simulink model "series"  (R2018b)
settings: Solver=ode1  StartTime=0.0  StopTime=t_stop  FixedStep=t_sample  RelTol=1e-3
values from neighbouring files (symbols this model uses):
  air_density_sea_level = 1.225    [hybrid_truck_script.m]
  battery_capacity = 24.5    [hybrid_truck_script.m]
  battery_efficiency = 0.8    [hybrid_truck_script.m]
  battery_max_power_flow = battery_v*battery_max_i    (= 23040)    [hybrid_truck_script.m]
  battery_no_of_modules = 15    [hybrid_truck_script.m]
  battery_SoC = 0.95    [hybrid_truck_script.m]
  constant_velocity = 60    [hybrid_truck_script.m]
  distance = 0.20    (= 0.2)    [hybrid_truck_script.m]
  drag_coeff = 0.65    [hybrid_truck_script.m]
  elevation = route.data(:,3)    [hybrid_truck_script.m]
  engine_optimum_rad = engine_rad(engine_optimum_index)    [hybrid_truck_script.m]
  engine_optimum_torque = max(engine_torque)    [hybrid_truck_script.m]
  frontal_area = 5.14    [hybrid_truck_script.m]
  fuel_map = (3.6e6/(engine_efficiency*fuel_LHV*fuel_density))*            (rps_axes'*torque_axes)    [hybrid_truck_script.m]
  g = 9.81    [hybrid_truck_script.m]
  gearRatio_differential = 4.263    [hybrid_truck_script.m]
  gradients = (pi/400).*route.data(:,5)    [hybrid_truck_script.m]
  momentOfInertia_engine = 2.55    [hybrid_truck_script.m]
  momentOfInertia_wheel = 2.5    [hybrid_truck_script.m]
  motor_efficiency = motor(1)    [hybrid_truck_script.m]
  mpsToKPH = 3.6    [hybrid_truck_script.m]
  radius_wheel = 0.46    [hybrid_truck_script.m]
  regeneration_efficiency = 0.75    [hybrid_truck_script.m]
  rolling_resistance = 0.008    [hybrid_truck_script.m]
  rps_axes = linspace(min(engine_rad),max(engine_rad),n)    [hybrid_truck_script.m]
  selection = number associated with the drive cycle (see    [drop_bars.m]    (also in hybrid_truck_script.m = listdlg('ListString', drive_cycle))
  t_sample = 0.1    [hybrid_truck_script.m]
  torque_axes = linspace(min(engine_torque),max(engine_torque),n)    [hybrid_truck_script.m]
  total_mass = mass_truck + mass_trailor    (= 39150)    [hybrid_truck_script.m]
libraries: dspstat3 x1, autolibshared x1
settings Model: Creator=tumisang  LastModifiedBy=tumisang

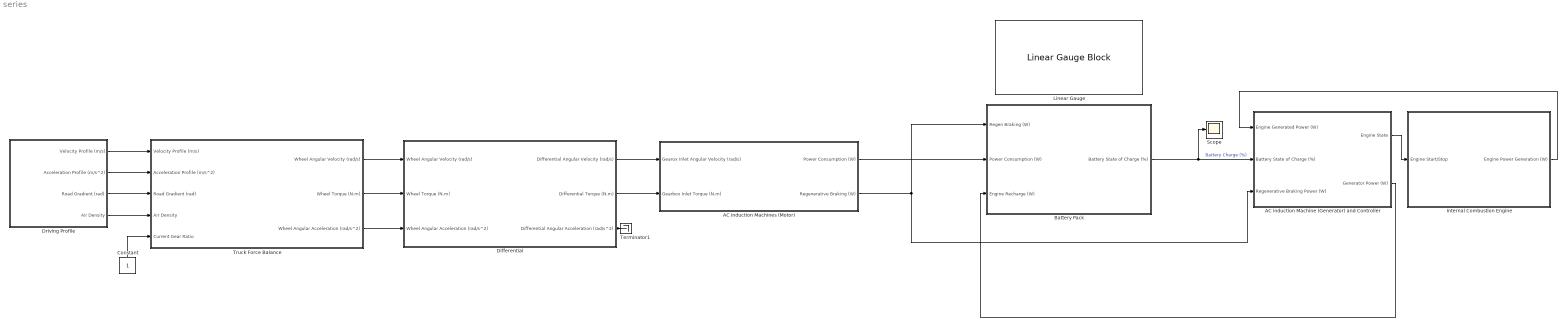
== system series ==
  " Battery Pack" : Subsystem
  AC Induction Machines (Motor) : Subsystem
  AC induction Machine (Generator) and Controller : Subsystem
  Constant : Constant
  Differential : Subsystem
  Driving Profile : Subsystem
  Internal Combustion Engine : Subsystem
  Linear Gauge : LinearGaugeBlock  WebBlockId=520
  Scope : Scope
  Terminator1 : Terminator
  Truck Force Balance : Subsystem
  wires:
  Differential/2(Differential Torque (N.m)) -> AC Induction Machines (Motor)/2(Gearbox Inlet Torque (N.m))
  AC Induction Machines (Motor)/2(Regenerative Braking (W)) -> " Battery Pack"/1(Regen Braking (W)), AC induction Machine (Generator) and Controller/3(Regenerative Braking Power (W))
  Internal Combustion Engine/1(Engine Power Generation (W)) -> AC induction Machine (Generator) and Controller/1(Engine Generated Power (W))
  AC induction Machine (Generator) and Controller/1(Engine State) -> Internal Combustion Engine/1(Engine Start/Stop)
  " Battery Pack"/1(Battery State of Charge (%)) -> AC induction Machine (Generator) and Controller/2(Battery State of Charge (%)), Scope/1  "Battery Charge (%)"
  AC Induction Machines (Motor)/1(Power Consumption (W)) -> " Battery Pack"/2(Power Consumption (W))
  AC induction Machine (Generator) and Controller/2(Generator Power (W)) -> " Battery Pack"/3(Engine Recharge (W))
  Truck Force Balance/3(Wheel Angular Acceleration (rad/s^2)) -> Differential/3(Wheel Angular Acceleration (rad/s^2))
  Truck Force Balance/2(Wheel Torque (N.m)) -> Differential/2(Wheel Torque (N.m))
  Truck Force Balance/1(Wheel Angular Velocity (rad/s)) -> Differential/1(Wheel Angular Velocity (rad/s))
  Constant/1 -> Truck Force Balance/5(Current Gear Ratio)
  Driving Profile/4(Air Density) -> Truck Force Balance/4(Air Density)
  Driving Profile/2(Acceleration Profile (m/s^2)) -> Truck Force Balance/2(Acceleration Profile (m/s^2))
  Driving Profile/1(Velocity Profile (m/s)) -> Truck Force Balance/1(Velocity Profile (m/s))
  Driving Profile/3(Road Gradient (rad)) -> Truck Force Balance/3(Road Gradient (rad))
  Differential/1(Differential Angular Velocity (rad/s)) -> AC Induction Machines (Motor)/1(Gearox Inlet Angular Velocity (rad/s))
  Differential/3(Differential Angular Acceleration (rad/s^2)) -> Terminator1/1

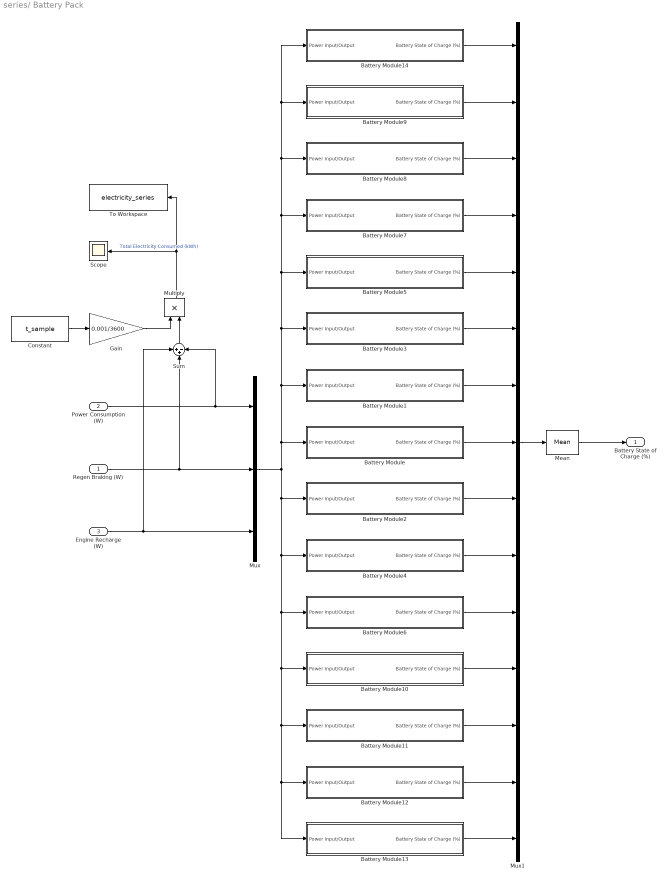
== system series/ Battery Pack ==
  Regen Braking (W) : Inport
  Power Consumption (W) : Inport  Port=2
  Engine Recharge (W) : Inport  Port=3
  Battery Module : Subsystem
  Battery Module1 : Subsystem
  Battery Module10 : Subsystem
  Battery Module11 : Subsystem
  Battery Module12 : Subsystem
  Battery Module13 : Subsystem
  Battery Module14 : Subsystem
  Battery Module2 : Subsystem
  Battery Module3 : Subsystem
  Battery Module4 : Subsystem
  Battery Module5 : Subsystem
  Battery Module6 : Subsystem
  Battery Module7 : Subsystem
  Battery Module8 : Subsystem
  Battery Module9 : Subsystem
  Constant : Constant  Value=t_sample
  Gain : Gain  Gain=0.001/3600
  Mean : dspstat3/Mean  run=off  InputProcessing=Columns as channels (frame based)  reset_popup=None  directionMode=Each column  dimension=1  roiEnable=off  roiType=Rectangles  roiPortion=Entire ROI  roiOutput=Individual statistics for each ROI  roiFlag=off  roundingMode=Floor  overflowMode=off  outputDataTypeStr=Inherit: Same as accumulator  outputMin=[]  outputMax=[]  outputLastDataTypeStr=Inherit: Same as accumulator
  Multiply : Product
  Mux : Mux  Inputs=3
  Mux1 : Mux  Inputs=15
  Scope : Scope
  Sum : Sum  Inputs=++-
  To Workspace : ToWorkspace  VariableName=electricity_series  SaveFormat=Timeseries  SampleTime=-1
  Battery State of Charge (%) : Outport
  wires:
  Mux/1 -> Battery Module11/1(Power Input/Output), Battery Module12/1(Power Input/Output), Battery Module13/1(Power Input/Output), Battery Module10/1(Power Input/Output), Battery Module6/1(Power Input/Output), Battery Module4/1(Power Input/Output), Battery Module2/1(Power Input/Output), Battery Module5/1(Power Input/Output), Battery Module7/1(Power Input/Output), Battery Module8/1(Power Input/Output), Battery Module9/1(Power Input/Output), Battery Module14/1(Power Input/Output), Battery Module3/1(Power Input/Output), Battery Module1/1(Power Input/Output), Battery Module/1(Power Input/Output)
  Battery Module1/1(Battery State of Charge (%)) -> Mux1/7
  Battery Module/1(Battery State of Charge (%)) -> Mux1/8
  Battery Module2/1(Battery State of Charge (%)) -> Mux1/9
  Battery Module4/1(Battery State of Charge (%)) -> Mux1/10
  Battery Module6/1(Battery State of Charge (%)) -> Mux1/11
  Battery Module3/1(Battery State of Charge (%)) -> Mux1/6
  Battery Module5/1(Battery State of Charge (%)) -> Mux1/5
  Battery Module7/1(Battery State of Charge (%)) -> Mux1/4
  Battery Module8/1(Battery State of Charge (%)) -> Mux1/3
  Battery Module9/1(Battery State of Charge (%)) -> Mux1/2
  Battery Module14/1(Battery State of Charge (%)) -> Mux1/1
  Battery Module10/1(Battery State of Charge (%)) -> Mux1/12
  Battery Module11/1(Battery State of Charge (%)) -> Mux1/13
  Battery Module12/1(Battery State of Charge (%)) -> Mux1/14
  Battery Module13/1(Battery State of Charge (%)) -> Mux1/15
  Mean/1 -> Battery State of Charge (%)/1
  Mux1/1 -> Mean/1
  Engine Recharge (W)/1 -> Mux/3, Sum/1
  Constant/1 -> Gain/1
  Power Consumption (W)/1 -> Mux/1, Sum/3
  Sum/1 -> Multiply/2
  Multiply/1 -> Scope/1, To Workspace/1  "Total Electricity Consumed (kWh)"
  Regen Braking (W)/1 -> Sum/2, Mux/2
  Gain/1 -> Multiply/1

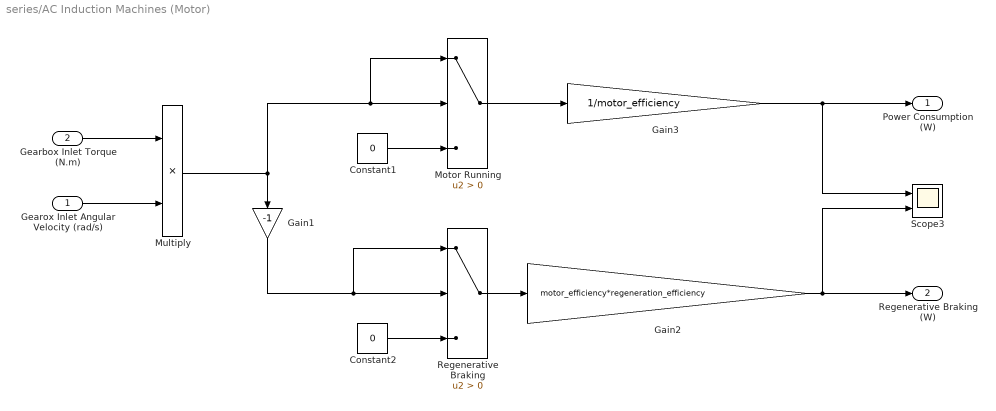
== system series/AC Induction Machines (Motor) ==
  Gearox Inlet Angular Velocity (rad/s) : Inport
  Gearbox Inlet Torque (N.m) : Inport  Port=2
  Constant1 : Constant  Value=0
  Constant2 : Constant  Value=0
  Gain1 : Gain  Gain=-1
  Gain2 : Gain  Gain=motor_efficiency*regeneration_efficiency
  Gain3 : Gain  Gain=1/motor_efficiency
  Motor Running : Switch  Criteria=u2 > Threshold
  Multiply : Product
  Regenerative Braking : Switch  Criteria=u2 > Threshold
  Scope3 : Scope  NumInputPorts=2
  Power Consumption (W) : Outport
  Regenerative Braking (W) : Outport  Port=2
  wires:
  Constant2/1 -> Regenerative Braking/3
  Constant1/1 -> Motor Running/3
  Gain2/1 -> Regenerative Braking (W)/1, Scope3/2
  Regenerative Braking/1 -> Gain2/1
  Multiply/1 -> Gain1/1, Motor Running/2, Motor Running/1
  Gain3/1 -> Power Consumption (W)/1, Scope3/1
  Gearox Inlet Angular Velocity (rad/s)/1 -> Multiply/2
  Gearbox Inlet Torque (N.m)/1 -> Multiply/1
  Motor Running/1 -> Gain3/1
  Gain1/1 -> Regenerative Braking/1, Regenerative Braking/2

== system series/AC induction Machine (Generator) and Controller ==
  Engine Generated Power (W) : Inport
  Battery State of Charge (%) : Inport  Port=2
  Regenerative Braking Power (W) : Inport  Port=3
  Engine On/Off Logic : Stateflow chart  TreatAsAtomicUnit=on
  Gain2 : Gain  Gain=regeneration_efficiency
  Engine State : Outport
  Generator Power (W) : Outport  Port=2
  wires:
  Gain2/1 -> Generator Power (W)/1
  Regenerative Braking Power (W)/1 -> Engine On/Off Logic/2(regen_power)
  Engine Generated Power (W)/1 -> Gain2/1
  Engine On/Off Logic/1(state) -> Engine State/1
  Battery State of Charge (%)/1 -> Engine On/Off Logic/1(battery_SoC)

== system series/Differential ==
  Wheel Angular Velocity (rad/s) : Inport
  Wheel Torque (N.m) : Inport  Port=2
  Wheel Angular Acceleration (rad/s^2) : Inport  Port=3
  Gain1 : Gain  Gain=1/gearRatio_differential
  Gain2 : Gain  Gain=gearRatio_differential
  Gain3 : Gain  Gain=gearRatio_differential
  Differential Angular Velocity (rad/s) : Outport
  Differential Torque (N.m) : Outport  Port=2
  Differential Angular Acceleration (rad/s^2) : Outport  Port=3
  wires:
  Gain2/1 -> Differential Angular Acceleration (rad/s^2)/1
  Gain3/1 -> Differential Angular Velocity (rad/s)/1
  Wheel Angular Acceleration (rad/s^2)/1 -> Gain2/1
  Wheel Torque (N.m)/1 -> Gain1/1
  Gain1/1 -> Differential Torque (N.m)/1
  Wheel Angular Velocity (rad/s)/1 -> Gain3/1

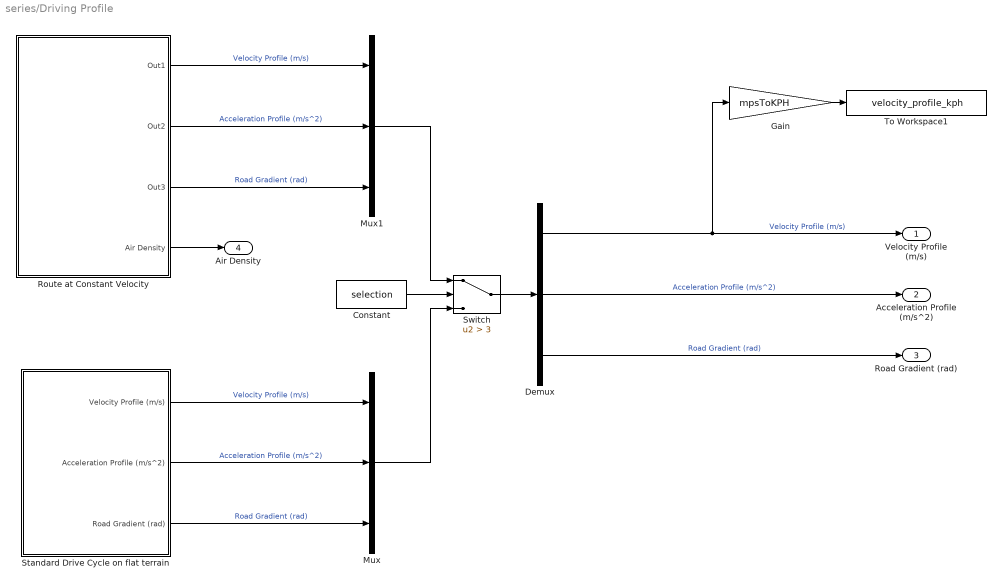
== system series/Driving Profile ==
  Constant : Constant  Value=selection
  Demux : Demux  Outputs=3
  Gain : Gain  Gain=mpsToKPH
  Mux : Mux  Inputs=3
  Mux1 : Mux  Inputs=3
  Route at Constant Velocity : Subsystem
  Standard Drive Cycle on flat terrain : Subsystem
  Switch : Switch  Criteria=u2 > Threshold  Threshold=3
  To Workspace1 : ToWorkspace  VariableName=velocity_profile_kph  SaveFormat=Timeseries  SampleTime=-1
  Velocity Profile (m/s) : Outport
  Acceleration Profile (m/s^2) : Outport  Port=2
  Road Gradient (rad) : Outport  Port=3
  Air Density : Outport  Port=4
  wires:
  Route at Constant Velocity/3(Out3) -> Mux1/3  "Road Gradient (rad)"
  Route at Constant Velocity/2(Out2) -> Mux1/2  "Acceleration Profile (m/s^2)"
  Demux/1 -> Velocity Profile (m/s)/1, Gain/1  "Velocity Profile (m/s)"
  Standard Drive Cycle on flat terrain/2(Acceleration Profile (m/s^2)) -> Mux/2  "Acceleration Profile (m/s^2)"
  Demux/2 -> Acceleration Profile (m/s^2)/1  "Acceleration Profile (m/s^2)"
  Standard Drive Cycle on flat terrain/3(Road Gradient (rad)) -> Mux/3  "Road Gradient (rad)"
  Demux/3 -> Road Gradient (rad)/1  "Road Gradient (rad)"
  Route at Constant Velocity/1(Out1) -> Mux1/1  "Velocity Profile (m/s)"
  Standard Drive Cycle on flat terrain/1(Velocity Profile (m/s)) -> Mux/1  "Velocity Profile (m/s)"
  Gain/1 -> To Workspace1/1
  Constant/1 -> Switch/2
  Switch/1 -> Demux/1
  Mux/1 -> Switch/3
  Mux1/1 -> Switch/1
  Route at Constant Velocity/4(Air Density) -> Air Density/1

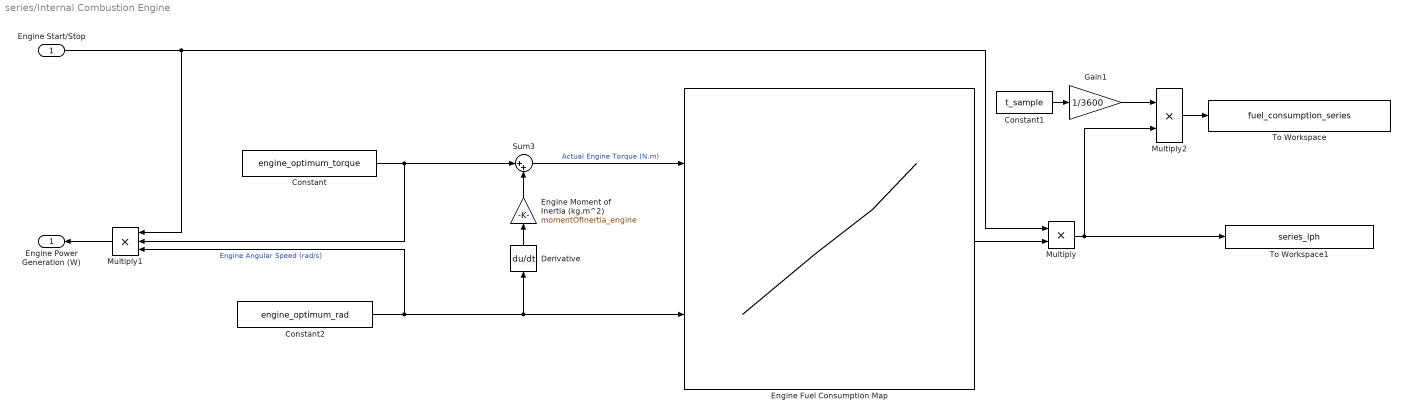
== system series/Internal Combustion Engine ==
  Engine Start/Stop : Inport
  Constant : Constant  Value=engine_optimum_torque
  Constant1 : Constant  Value=t_sample
  Constant2 : Constant  Value=engine_optimum_rad
  Derivative : Derivative  CoefficientInTFapproximation=0
  Engine Fuel Consumption Map : Lookup_n-D  BreakpointsForDimension1=torque_axes  BreakpointsForDimension2=rps_axes  Table=fuel_map  InternalRulePriority=Speed  RndMeth=Simplest  InputSameDT=on
  Engine Moment of Inertia (kg.m^2) : Gain  Gain=momentOfInertia_engine
  Gain1 : Gain  Gain=1/3600
  Multiply : Product
  Multiply1 : Product  Inputs=3
  Multiply2 : Product
  Sum3 : Sum  Inputs=|++
  To Workspace : ToWorkspace  VariableName=fuel_consumption_series  SaveFormat=Timeseries  SampleTime=-1
  To Workspace1 : ToWorkspace  VariableName=series_lph  SaveFormat=Timeseries  SampleTime=-1
  Engine Power Generation (W) : Outport
  wires:
  Constant2/1 -> Engine Fuel Consumption Map/2, Derivative/1, Multiply1/3  "Engine Angular Speed (rad/s)"
  Sum3/1 -> Engine Fuel Consumption Map/1  "Actual Engine Torque (N.m)"
  Engine Moment of Inertia (kg.m^2)/1 -> Sum3/2
  Engine Fuel Consumption Map/1 -> Multiply/2
  Derivative/1 -> Engine Moment of Inertia (kg.m^2)/1
  Constant/1 -> Multiply1/2, Sum3/1
  Engine Start/Stop/1 -> Multiply/1, Multiply1/1
  Multiply1/1 -> Engine Power Generation (W)/1
  Multiply/1 -> To Workspace1/1, Multiply2/2
  Multiply2/1 -> To Workspace/1
  Gain1/1 -> Multiply2/1
  Constant1/1 -> Gain1/1

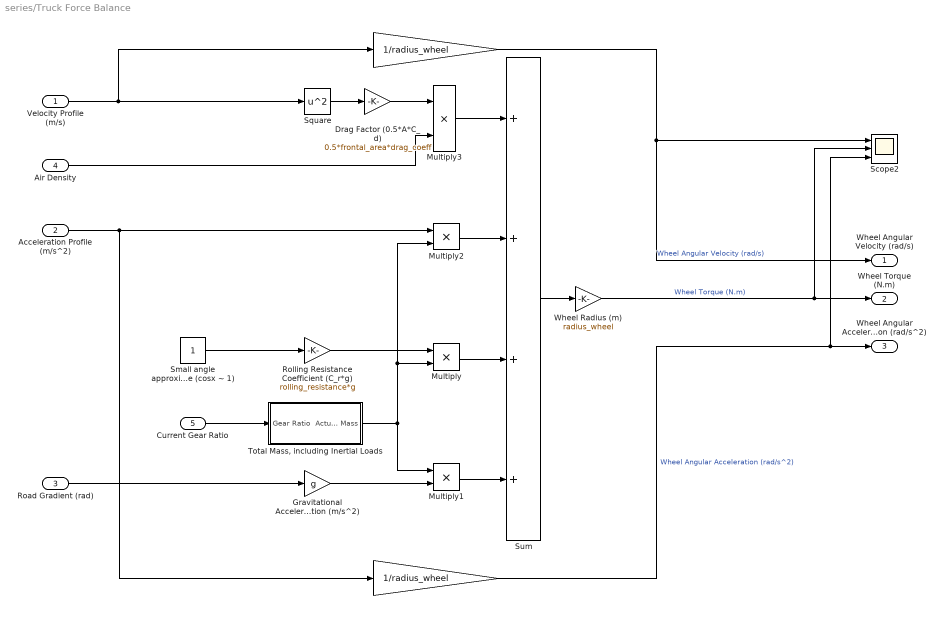
== system series/Truck Force Balance ==
  Velocity Profile (m/s) : Inport
  Acceleration Profile (m/s^2) : Inport  Port=2
  Road Gradient (rad) : Inport  Port=3
  Air Density : Inport  Port=4
  Current Gear Ratio : Inport  Port=5
  " " : Gain  Gain=1/radius_wheel
  " " : Gain  Gain=1/radius_wheel
  Drag Factor (0.5*A*C_d) : Gain  Gain=0.5*frontal_area*drag_coeff
  Gravitational Acceleration (m/s^2) : Gain  Gain=g
  Multiply{,1..3} (4 alike) : Product
  Rolling Resistance Coefficient (C_r*g) : Gain  Gain=rolling_resistance*g
  Scope2 : Scope  NumInputPorts=3
  Small angle approximation for cosine (cosx ~ 1) : Constant
  Square : Math  Operator=square  SaturateOnIntegerOverflow=on
  Sum : Sum  Inputs=++++
  "Total Mass, including Inertial Loads" : Subsystem
  Wheel Radius (m) : Gain  Gain=radius_wheel
  Wheel Angular Velocity (rad/s) : Outport
  Wheel Torque (N.m) : Outport  Port=2
  Wheel Angular Acceleration (rad/s^2) : Outport  Port=3
  wires:
  Square/1 -> Drag Factor (0.5*A*C_d)/1
  Drag Factor (0.5*A*C_d)/1 -> Multiply3/1
  Road Gradient (rad)/1 -> Gravitational Acceleration (m/s^2)/1
  Gravitational Acceleration (m/s^2)/1 -> Multiply1/2
  Velocity Profile (m/s)/1 -> Square/1, " "/1
  Rolling Resistance Coefficient (C_r*g)/1 -> Multiply/1
  Sum/1 -> Wheel Radius (m)/1
  Wheel Radius (m)/1 -> Wheel Torque (N.m)/1, Scope2/2  "Wheel Torque (N.m)"
  " "/1 -> Scope2/3, Wheel Angular Acceleration (rad/s^2)/1  "Wheel Angular Acceleration (rad/s^2)"
  " "/1 -> Wheel Angular Velocity (rad/s)/1, Scope2/1  "Wheel Angular Velocity (rad/s)"
  Multiply2/1 -> Sum/2
  Small angle approximation for cosine (cosx ~ 1)/1 -> Rolling Resistance Coefficient (C_r*g)/1
  Acceleration Profile (m/s^2)/1 -> " "/1, Multiply2/1
  Current Gear Ratio/1 -> "Total Mass, including Inertial Loads"/1("Gear Ratio ")
  "Total Mass, including Inertial Loads"/1(Actual Mass) -> Multiply1/1, Multiply2/2, Multiply/2
  Multiply/1 -> Sum/3
  Multiply1/1 -> Sum/4
  Air Density/1 -> Multiply3/2
  Multiply3/1 -> Sum/1

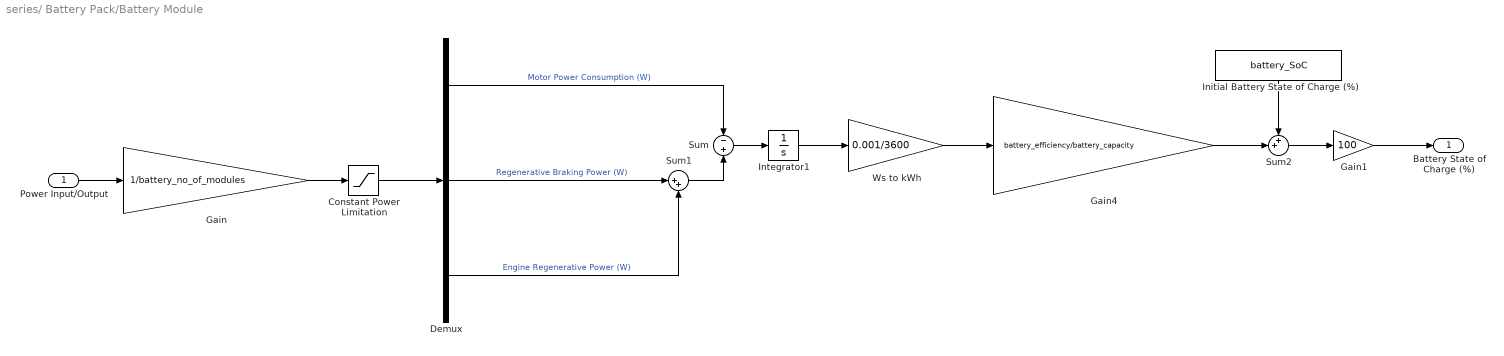
== system series/ Battery Pack/Battery Module ==
  Power Input/Output : Inport
  Constant Power Limitation : Saturate  UpperLimit=battery_max_power_flow  LowerLimit=0
  Demux : Demux  Outputs=3
  Gain : Gain  Gain=1/battery_no_of_modules
  Gain1 : Gain  Gain=100
  Gain4 : Gain  Gain=battery_efficiency/battery_capacity
  Initial Battery State of Charge (%) : Constant  Value=battery_SoC
  Integrator1 : Integrator
  Sum : Sum  Inputs=-+
  Sum1 : Sum  Inputs=|++
  Sum2 : Sum  Inputs=++|
  Ws to kWh : Gain  Gain=0.001/3600
  Battery State of Charge (%) : Outport
  wires:
  Sum/1 -> Integrator1/1
  Ws to kWh/1 -> Gain4/1
  Initial Battery State of Charge (%)/1 -> Sum2/1
  Sum2/1 -> Gain1/1
  Gain1/1 -> Battery State of Charge (%)/1
  Sum1/1 -> Sum/2
  Integrator1/1 -> Ws to kWh/1
  Gain4/1 -> Sum2/2
  Demux/3 -> Sum1/2  "Engine Regenerative Power (W)"
  Demux/2 -> Sum1/1  "Regenerative Braking Power (W)"
  Demux/1 -> Sum/1  "Motor Power Consumption (W)"
  Gain/1 -> Constant Power Limitation/1
  Power Input/Output/1 -> Gain/1
  Constant Power Limitation/1 -> Demux/1

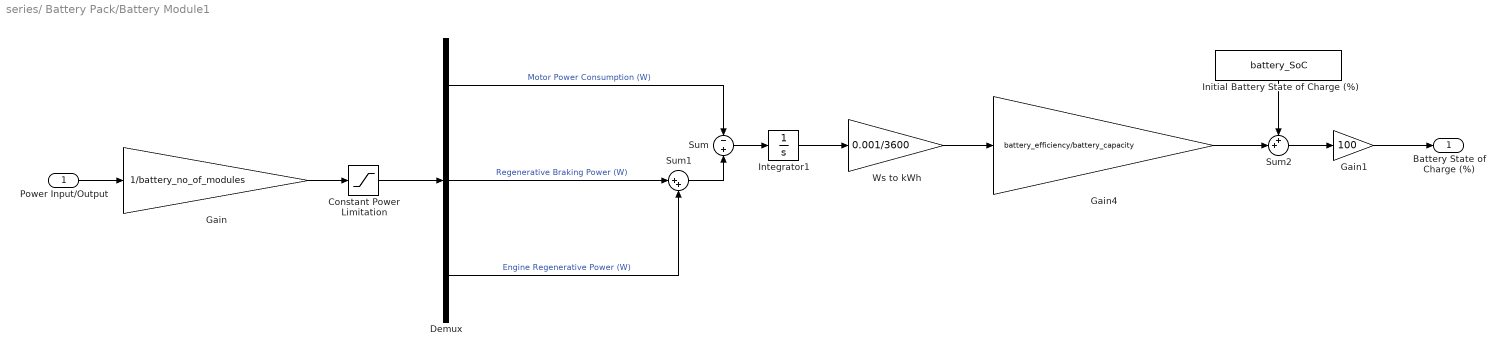
== system series/ Battery Pack/Battery Module1 ==
  Power Input/Output : Inport
  Constant Power Limitation : Saturate  UpperLimit=battery_max_power_flow  LowerLimit=0
  Demux : Demux  Outputs=3
  Gain : Gain  Gain=1/battery_no_of_modules
  Gain1 : Gain  Gain=100
  Gain4 : Gain  Gain=battery_efficiency/battery_capacity
  Initial Battery State of Charge (%) : Constant  Value=battery_SoC
  Integrator1 : Integrator
  Sum : Sum  Inputs=-+
  Sum1 : Sum  Inputs=|++
  Sum2 : Sum  Inputs=++|
  Ws to kWh : Gain  Gain=0.001/3600
  Battery State of Charge (%) : Outport
  wires:
  Constant Power Limitation/1 -> Demux/1
  Power Input/Output/1 -> Gain/1
  Gain/1 -> Constant Power Limitation/1
  Demux/1 -> Sum/1  "Motor Power Consumption (W)"
  Demux/2 -> Sum1/1  "Regenerative Braking Power (W)"
  Demux/3 -> Sum1/2  "Engine Regenerative Power (W)"
  Gain4/1 -> Sum2/2
  Integrator1/1 -> Ws to kWh/1
  Sum1/1 -> Sum/2
  Gain1/1 -> Battery State of Charge (%)/1
  Sum2/1 -> Gain1/1
  Initial Battery State of Charge (%)/1 -> Sum2/1
  Ws to kWh/1 -> Gain4/1
  Sum/1 -> Integrator1/1

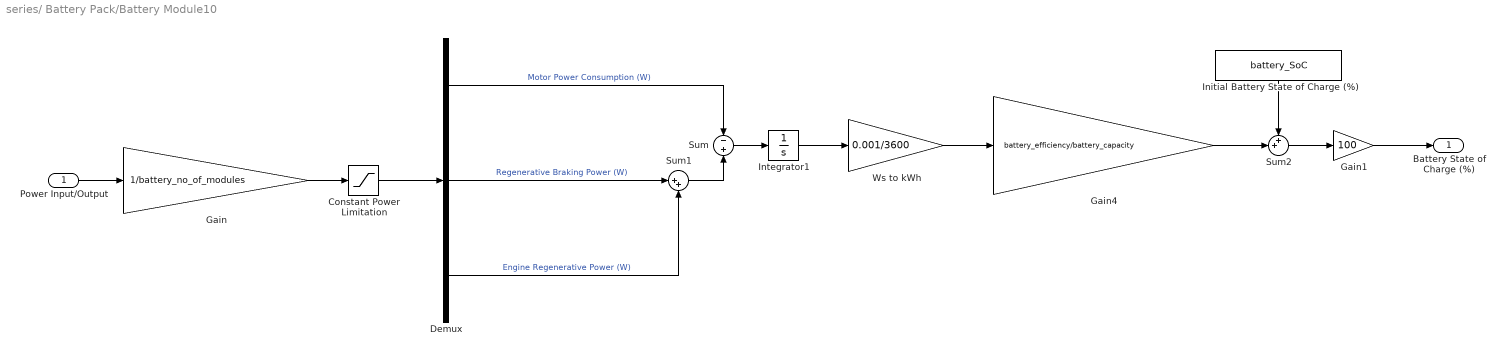
== system series/ Battery Pack/Battery Module10 ==
  Power Input/Output : Inport
  Constant Power Limitation : Saturate  UpperLimit=battery_max_power_flow  LowerLimit=0
  Demux : Demux  Outputs=3
  Gain : Gain  Gain=1/battery_no_of_modules
  Gain1 : Gain  Gain=100
  Gain4 : Gain  Gain=battery_efficiency/battery_capacity
  Initial Battery State of Charge (%) : Constant  Value=battery_SoC
  Integrator1 : Integrator
  Sum : Sum  Inputs=-+
  Sum1 : Sum  Inputs=|++
  Sum2 : Sum  Inputs=++|
  Ws to kWh : Gain  Gain=0.001/3600
  Battery State of Charge (%) : Outport
  wires:
  Constant Power Limitation/1 -> Demux/1
  Power Input/Output/1 -> Gain/1
  Gain/1 -> Constant Power Limitation/1
  Demux/1 -> Sum/1  "Motor Power Consumption (W)"
  Demux/2 -> Sum1/1  "Regenerative Braking Power (W)"
  Demux/3 -> Sum1/2  "Engine Regenerative Power (W)"
  Gain4/1 -> Sum2/2
  Integrator1/1 -> Ws to kWh/1
  Sum1/1 -> Sum/2
  Gain1/1 -> Battery State of Charge (%)/1
  Sum2/1 -> Gain1/1
  Initial Battery State of Charge (%)/1 -> Sum2/1
  Ws to kWh/1 -> Gain4/1
  Sum/1 -> Integrator1/1

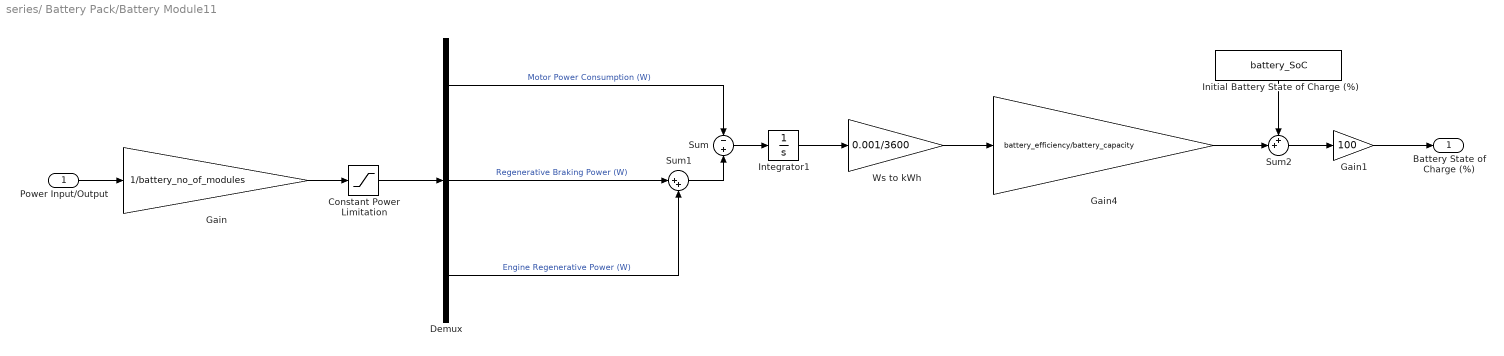
== system series/ Battery Pack/Battery Module11 ==
  Power Input/Output : Inport
  Constant Power Limitation : Saturate  UpperLimit=battery_max_power_flow  LowerLimit=0
  Demux : Demux  Outputs=3
  Gain : Gain  Gain=1/battery_no_of_modules
  Gain1 : Gain  Gain=100
  Gain4 : Gain  Gain=battery_efficiency/battery_capacity
  Initial Battery State of Charge (%) : Constant  Value=battery_SoC
  Integrator1 : Integrator
  Sum : Sum  Inputs=-+
  Sum1 : Sum  Inputs=|++
  Sum2 : Sum  Inputs=++|
  Ws to kWh : Gain  Gain=0.001/3600
  Battery State of Charge (%) : Outport
  wires:
  Sum/1 -> Integrator1/1
  Ws to kWh/1 -> Gain4/1
  Initial Battery State of Charge (%)/1 -> Sum2/1
  Sum2/1 -> Gain1/1
  Gain1/1 -> Battery State of Charge (%)/1
  Sum1/1 -> Sum/2
  Integrator1/1 -> Ws to kWh/1
  Gain4/1 -> Sum2/2
  Demux/3 -> Sum1/2  "Engine Regenerative Power (W)"
  Demux/2 -> Sum1/1  "Regenerative Braking Power (W)"
  Demux/1 -> Sum/1  "Motor Power Consumption (W)"
  Gain/1 -> Constant Power Limitation/1
  Power Input/Output/1 -> Gain/1
  Constant Power Limitation/1 -> Demux/1

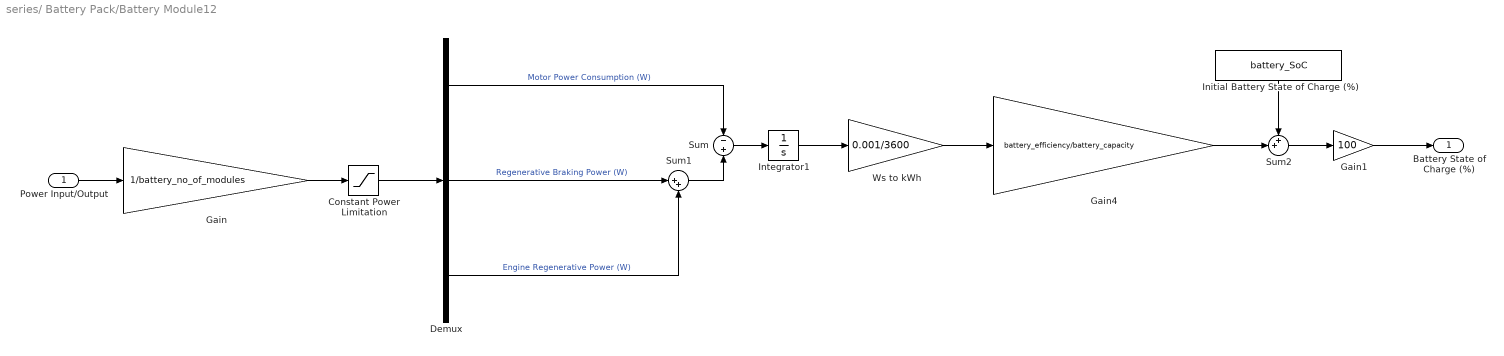
== system series/ Battery Pack/Battery Module12 ==
  Power Input/Output : Inport
  Constant Power Limitation : Saturate  UpperLimit=battery_max_power_flow  LowerLimit=0
  Demux : Demux  Outputs=3
  Gain : Gain  Gain=1/battery_no_of_modules
  Gain1 : Gain  Gain=100
  Gain4 : Gain  Gain=battery_efficiency/battery_capacity
  Initial Battery State of Charge (%) : Constant  Value=battery_SoC
  Integrator1 : Integrator
  Sum : Sum  Inputs=-+
  Sum1 : Sum  Inputs=|++
  Sum2 : Sum  Inputs=++|
  Ws to kWh : Gain  Gain=0.001/3600
  Battery State of Charge (%) : Outport
  wires:
  Constant Power Limitation/1 -> Demux/1
  Power Input/Output/1 -> Gain/1
  Gain/1 -> Constant Power Limitation/1
  Demux/1 -> Sum/1  "Motor Power Consumption (W)"
  Demux/2 -> Sum1/1  "Regenerative Braking Power (W)"
  Demux/3 -> Sum1/2  "Engine Regenerative Power (W)"
  Gain4/1 -> Sum2/2
  Integrator1/1 -> Ws to kWh/1
  Sum1/1 -> Sum/2
  Gain1/1 -> Battery State of Charge (%)/1
  Sum2/1 -> Gain1/1
  Initial Battery State of Charge (%)/1 -> Sum2/1
  Ws to kWh/1 -> Gain4/1
  Sum/1 -> Integrator1/1

== system series/ Battery Pack/Battery Module13 ==
  Power Input/Output : Inport
  Constant Power Limitation : Saturate  UpperLimit=battery_max_power_flow  LowerLimit=0
  Demux : Demux  Outputs=3
  Gain : Gain  Gain=1/battery_no_of_modules
  Gain1 : Gain  Gain=100
  Gain4 : Gain  Gain=battery_efficiency/battery_capacity
  Initial Battery State of Charge (%) : Constant  Value=battery_SoC
  Integrator1 : Integrator
  Sum : Sum  Inputs=-+
  Sum1 : Sum  Inputs=|++
  Sum2 : Sum  Inputs=++|
  Ws to kWh : Gain  Gain=0.001/3600
  Battery State of Charge (%) : Outport
  wires:
  Sum/1 -> Integrator1/1
  Ws to kWh/1 -> Gain4/1
  Initial Battery State of Charge (%)/1 -> Sum2/1
  Sum2/1 -> Gain1/1
  Gain1/1 -> Battery State of Charge (%)/1
  Sum1/1 -> Sum/2
  Integrator1/1 -> Ws to kWh/1
  Gain4/1 -> Sum2/2
  Demux/3 -> Sum1/2  "Engine Regenerative Power (W)"
  Demux/2 -> Sum1/1  "Regenerative Braking Power (W)"
  Demux/1 -> Sum/1  "Motor Power Consumption (W)"
  Gain/1 -> Constant Power Limitation/1
  Power Input/Output/1 -> Gain/1
  Constant Power Limitation/1 -> Demux/1

== system series/ Battery Pack/Battery Module14 ==
  Power Input/Output : Inport
  Constant Power Limitation : Saturate  UpperLimit=battery_max_power_flow  LowerLimit=0
  Demux : Demux  Outputs=3
  Gain : Gain  Gain=1/battery_no_of_modules
  Gain1 : Gain  Gain=100
  Gain4 : Gain  Gain=battery_efficiency/battery_capacity
  Initial Battery State of Charge (%) : Constant  Value=battery_SoC
  Integrator1 : Integrator
  Sum : Sum  Inputs=-+
  Sum1 : Sum  Inputs=|++
  Sum2 : Sum  Inputs=++|
  Ws to kWh : Gain  Gain=0.001/3600
  Battery State of Charge (%) : Outport
  wires:
  Constant Power Limitation/1 -> Demux/1
  Power Input/Output/1 -> Gain/1
  Gain/1 -> Constant Power Limitation/1
  Demux/1 -> Sum/1  "Motor Power Consumption (W)"
  Demux/2 -> Sum1/1  "Regenerative Braking Power (W)"
  Demux/3 -> Sum1/2  "Engine Regenerative Power (W)"
  Gain4/1 -> Sum2/2
  Integrator1/1 -> Ws to kWh/1
  Sum1/1 -> Sum/2
  Gain1/1 -> Battery State of Charge (%)/1
  Sum2/1 -> Gain1/1
  Initial Battery State of Charge (%)/1 -> Sum2/1
  Ws to kWh/1 -> Gain4/1
  Sum/1 -> Integrator1/1

== system series/ Battery Pack/Battery Module2 ==
  Power Input/Output : Inport
  Constant Power Limitation : Saturate  UpperLimit=battery_max_power_flow  LowerLimit=0
  Demux : Demux  Outputs=3
  Gain : Gain  Gain=1/battery_no_of_modules
  Gain1 : Gain  Gain=100
  Gain4 : Gain  Gain=battery_efficiency/battery_capacity
  Initial Battery State of Charge (%) : Constant  Value=battery_SoC
  Integrator1 : Integrator
  Sum : Sum  Inputs=-+
  Sum1 : Sum  Inputs=|++
  Sum2 : Sum  Inputs=++|
  Ws to kWh : Gain  Gain=0.001/3600
  Battery State of Charge (%) : Outport
  wires:
  Constant Power Limitation/1 -> Demux/1
  Power Input/Output/1 -> Gain/1
  Gain/1 -> Constant Power Limitation/1
  Demux/1 -> Sum/1  "Motor Power Consumption (W)"
  Demux/2 -> Sum1/1  "Regenerative Braking Power (W)"
  Demux/3 -> Sum1/2  "Engine Regenerative Power (W)"
  Gain4/1 -> Sum2/2
  Integrator1/1 -> Ws to kWh/1
  Sum1/1 -> Sum/2
  Gain1/1 -> Battery State of Charge (%)/1
  Sum2/1 -> Gain1/1
  Initial Battery State of Charge (%)/1 -> Sum2/1
  Ws to kWh/1 -> Gain4/1
  Sum/1 -> Integrator1/1

== system series/ Battery Pack/Battery Module3 ==
  Power Input/Output : Inport
  Constant Power Limitation : Saturate  UpperLimit=battery_max_power_flow  LowerLimit=0
  Demux : Demux  Outputs=3
  Gain : Gain  Gain=1/battery_no_of_modules
  Gain1 : Gain  Gain=100
  Gain4 : Gain  Gain=battery_efficiency/battery_capacity
  Initial Battery State of Charge (%) : Constant  Value=battery_SoC
  Integrator1 : Integrator
  Sum : Sum  Inputs=-+
  Sum1 : Sum  Inputs=|++
  Sum2 : Sum  Inputs=++|
  Ws to kWh : Gain  Gain=0.001/3600
  Battery State of Charge (%) : Outport
  wires:
  Sum/1 -> Integrator1/1
  Ws to kWh/1 -> Gain4/1
  Initial Battery State of Charge (%)/1 -> Sum2/1
  Sum2/1 -> Gain1/1
  Gain1/1 -> Battery State of Charge (%)/1
  Sum1/1 -> Sum/2
  Integrator1/1 -> Ws to kWh/1
  Gain4/1 -> Sum2/2
  Demux/3 -> Sum1/2  "Engine Regenerative Power (W)"
  Demux/2 -> Sum1/1  "Regenerative Braking Power (W)"
  Demux/1 -> Sum/1  "Motor Power Consumption (W)"
  Gain/1 -> Constant Power Limitation/1
  Power Input/Output/1 -> Gain/1
  Constant Power Limitation/1 -> Demux/1

== system series/ Battery Pack/Battery Module4 ==
  Power Input/Output : Inport
  Constant Power Limitation : Saturate  UpperLimit=battery_max_power_flow  LowerLimit=0
  Demux : Demux  Outputs=3
  Gain : Gain  Gain=1/battery_no_of_modules
  Gain1 : Gain  Gain=100
  Gain4 : Gain  Gain=battery_efficiency/battery_capacity
  Initial Battery State of Charge (%) : Constant  Value=battery_SoC
  Integrator1 : Integrator
  Sum : Sum  Inputs=-+
  Sum1 : Sum  Inputs=|++
  Sum2 : Sum  Inputs=++|
  Ws to kWh : Gain  Gain=0.001/3600
  Battery State of Charge (%) : Outport
  wires:
  Constant Power Limitation/1 -> Demux/1
  Power Input/Output/1 -> Gain/1
  Gain/1 -> Constant Power Limitation/1
  Demux/1 -> Sum/1  "Motor Power Consumption (W)"
  Demux/2 -> Sum1/1  "Regenerative Braking Power (W)"
  Demux/3 -> Sum1/2  "Engine Regenerative Power (W)"
  Gain4/1 -> Sum2/2
  Integrator1/1 -> Ws to kWh/1
  Sum1/1 -> Sum/2
  Gain1/1 -> Battery State of Charge (%)/1
  Sum2/1 -> Gain1/1
  Initial Battery State of Charge (%)/1 -> Sum2/1
  Ws to kWh/1 -> Gain4/1
  Sum/1 -> Integrator1/1

== system series/ Battery Pack/Battery Module5 ==
  Power Input/Output : Inport
  Constant Power Limitation : Saturate  UpperLimit=battery_max_power_flow  LowerLimit=0
  Demux : Demux  Outputs=3
  Gain : Gain  Gain=1/battery_no_of_modules
  Gain1 : Gain  Gain=100
  Gain4 : Gain  Gain=battery_efficiency/battery_capacity
  Initial Battery State of Charge (%) : Constant  Value=battery_SoC
  Integrator1 : Integrator
  Sum : Sum  Inputs=-+
  Sum1 : Sum  Inputs=|++
  Sum2 : Sum  Inputs=++|
  Ws to kWh : Gain  Gain=0.001/3600
  Battery State of Charge (%) : Outport
  wires:
  Constant Power Limitation/1 -> Demux/1
  Power Input/Output/1 -> Gain/1
  Gain/1 -> Constant Power Limitation/1
  Demux/1 -> Sum/1  "Motor Power Consumption (W)"
  Demux/2 -> Sum1/1  "Regenerative Braking Power (W)"
  Demux/3 -> Sum1/2  "Engine Regenerative Power (W)"
  Gain4/1 -> Sum2/2
  Integrator1/1 -> Ws to kWh/1
  Sum1/1 -> Sum/2
  Gain1/1 -> Battery State of Charge (%)/1
  Sum2/1 -> Gain1/1
  Initial Battery State of Charge (%)/1 -> Sum2/1
  Ws to kWh/1 -> Gain4/1
  Sum/1 -> Integrator1/1

== system series/ Battery Pack/Battery Module6 ==
  Power Input/Output : Inport
  Constant Power Limitation : Saturate  UpperLimit=battery_max_power_flow  LowerLimit=0
  Demux : Demux  Outputs=3
  Gain : Gain  Gain=1/battery_no_of_modules
  Gain1 : Gain  Gain=100
  Gain4 : Gain  Gain=battery_efficiency/battery_capacity
  Initial Battery State of Charge (%) : Constant  Value=battery_SoC
  Integrator1 : Integrator
  Sum : Sum  Inputs=-+
  Sum1 : Sum  Inputs=|++
  Sum2 : Sum  Inputs=++|
  Ws to kWh : Gain  Gain=0.001/3600
  Battery State of Charge (%) : Outport
  wires:
  Sum/1 -> Integrator1/1
  Ws to kWh/1 -> Gain4/1
  Initial Battery State of Charge (%)/1 -> Sum2/1
  Sum2/1 -> Gain1/1
  Gain1/1 -> Battery State of Charge (%)/1
  Sum1/1 -> Sum/2
  Integrator1/1 -> Ws to kWh/1
  Gain4/1 -> Sum2/2
  Demux/3 -> Sum1/2  "Engine Regenerative Power (W)"
  Demux/2 -> Sum1/1  "Regenerative Braking Power (W)"
  Demux/1 -> Sum/1  "Motor Power Consumption (W)"
  Gain/1 -> Constant Power Limitation/1
  Power Input/Output/1 -> Gain/1
  Constant Power Limitation/1 -> Demux/1

== system series/ Battery Pack/Battery Module7 ==
  Power Input/Output : Inport
  Constant Power Limitation : Saturate  UpperLimit=battery_max_power_flow  LowerLimit=0
  Demux : Demux  Outputs=3
  Gain : Gain  Gain=1/battery_no_of_modules
  Gain1 : Gain  Gain=100
  Gain4 : Gain  Gain=battery_efficiency/battery_capacity
  Initial Battery State of Charge (%) : Constant  Value=battery_SoC
  Integrator1 : Integrator
  Sum : Sum  Inputs=-+
  Sum1 : Sum  Inputs=|++
  Sum2 : Sum  Inputs=++|
  Ws to kWh : Gain  Gain=0.001/3600
  Battery State of Charge (%) : Outport
  wires:
  Sum/1 -> Integrator1/1
  Ws to kWh/1 -> Gain4/1
  Initial Battery State of Charge (%)/1 -> Sum2/1
  Sum2/1 -> Gain1/1
  Gain1/1 -> Battery State of Charge (%)/1
  Sum1/1 -> Sum/2
  Integrator1/1 -> Ws to kWh/1
  Gain4/1 -> Sum2/2
  Demux/3 -> Sum1/2  "Engine Regenerative Power (W)"
  Demux/2 -> Sum1/1  "Regenerative Braking Power (W)"
  Demux/1 -> Sum/1  "Motor Power Consumption (W)"
  Gain/1 -> Constant Power Limitation/1
  Power Input/Output/1 -> Gain/1
  Constant Power Limitation/1 -> Demux/1

== system series/ Battery Pack/Battery Module8 ==
  Power Input/Output : Inport
  Constant Power Limitation : Saturate  UpperLimit=battery_max_power_flow  LowerLimit=0
  Demux : Demux  Outputs=3
  Gain : Gain  Gain=1/battery_no_of_modules
  Gain1 : Gain  Gain=100
  Gain4 : Gain  Gain=battery_efficiency/battery_capacity
  Initial Battery State of Charge (%) : Constant  Value=battery_SoC
  Integrator1 : Integrator
  Sum : Sum  Inputs=-+
  Sum1 : Sum  Inputs=|++
  Sum2 : Sum  Inputs=++|
  Ws to kWh : Gain  Gain=0.001/3600
  Battery State of Charge (%) : Outport
  wires:
  Constant Power Limitation/1 -> Demux/1
  Power Input/Output/1 -> Gain/1
  Gain/1 -> Constant Power Limitation/1
  Demux/1 -> Sum/1  "Motor Power Consumption (W)"
  Demux/2 -> Sum1/1  "Regenerative Braking Power (W)"
  Demux/3 -> Sum1/2  "Engine Regenerative Power (W)"
  Gain4/1 -> Sum2/2
  Integrator1/1 -> Ws to kWh/1
  Sum1/1 -> Sum/2
  Gain1/1 -> Battery State of Charge (%)/1
  Sum2/1 -> Gain1/1
  Initial Battery State of Charge (%)/1 -> Sum2/1
  Ws to kWh/1 -> Gain4/1
  Sum/1 -> Integrator1/1

== system series/ Battery Pack/Battery Module9 ==
  Power Input/Output : Inport
  Constant Power Limitation : Saturate  UpperLimit=battery_max_power_flow  LowerLimit=0
  Demux : Demux  Outputs=3
  Gain : Gain  Gain=1/battery_no_of_modules
  Gain1 : Gain  Gain=100
  Gain4 : Gain  Gain=battery_efficiency/battery_capacity
  Initial Battery State of Charge (%) : Constant  Value=battery_SoC
  Integrator1 : Integrator
  Sum : Sum  Inputs=-+
  Sum1 : Sum  Inputs=|++
  Sum2 : Sum  Inputs=++|
  Ws to kWh : Gain  Gain=0.001/3600
  Battery State of Charge (%) : Outport
  wires:
  Sum/1 -> Integrator1/1
  Ws to kWh/1 -> Gain4/1
  Initial Battery State of Charge (%)/1 -> Sum2/1
  Sum2/1 -> Gain1/1
  Gain1/1 -> Battery State of Charge (%)/1
  Sum1/1 -> Sum/2
  Integrator1/1 -> Ws to kWh/1
  Gain4/1 -> Sum2/2
  Demux/3 -> Sum1/2  "Engine Regenerative Power (W)"
  Demux/2 -> Sum1/1  "Regenerative Braking Power (W)"
  Demux/1 -> Sum/1  "Motor Power Consumption (W)"
  Gain/1 -> Constant Power Limitation/1
  Power Input/Output/1 -> Gain/1
  Constant Power Limitation/1 -> Demux/1

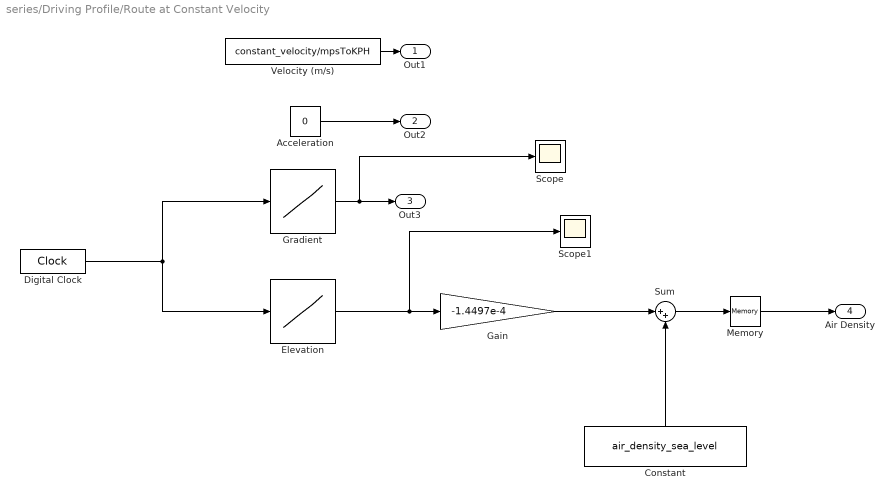
== system series/Driving Profile/Route at Constant Velocity ==
  Acceleration : Constant  Value=0
  Constant : Constant  Value=air_density_sea_level
  Digital Clock : DigitalClock
  Elevation : Lookup_n-D  NumberOfTableDimensions=1  BreakpointsSpecification=Even spacing  BreakpointsForDimension1=distance(:,1)  Table=elevation  InternalRulePriority=Speed  RndMeth=Simplest  InputSameDT=on
  Gain : Gain  Gain=-1.4497e-4
  Gradient : Lookup_n-D  NumberOfTableDimensions=1  LookupTableObject=gradients  BreakpointsSpecification=Even spacing  BreakpointsForDimension1=linspace(0, max(distance), length(distance))  BreakpointsForDimension1FirstPoint=0  Table=gradients  InternalRulePriority=Speed  RndMeth=Simplest  InputSameDT=on
  Memory : Memory  InitialCondition=air_density_sea_level
  Scope : Scope
  Scope1 : Scope
  Sum : Sum  Inputs=|++
  Velocity (m/s) : Constant  Value=constant_velocity/mpsToKPH
  Out1 : Outport
  Out2 : Outport  Port=2
  Out3 : Outport  Port=3
  Air Density : Outport  Port=4
  wires:
  Acceleration/1 -> Out2/1
  Velocity (m/s)/1 -> Out1/1
  Elevation/1 -> Scope1/1, Gain/1
  Constant/1 -> Sum/2
  Gradient/1 -> Scope/1, Out3/1
  Sum/1 -> Memory/1
  Gain/1 -> Sum/1
  Memory/1 -> Air Density/1
  Digital Clock/1 -> Gradient/1, Elevation/1

== system series/Driving Profile/Standard Drive Cycle on flat terrain ==
  Drive Cycle Source : autolibshared/Drive Cycle Source  cycleVar=Heavy Heavy-Duty Diesel Truck (HHDDT) - Cruise Mode  fileVar=cycleFTP75.mat  tfinal="2083  seconds"  cycleRepeat=off  outAccPort=on  outGearPort=off  gearList=No gear data  t_wot1=5  xdot_woto=0  xdot_wot1=30  t_wot2=20  xdot_wot2=0  t_wotend=30  srcUnit=m/s  outUnit=m/s  srcAccUnit=m/s/s  outAccUnit=m/s^2  dt=t_sample  aMode=2
      settings: SourceProductName=Powertrain Blockset  SourceProductBaseCode=PW
  Road Gradient (rad) : Constant  Value=0
  Velocity Profile (m/s) : Outport
  Acceleration Profile (m/s^2) : Outport  Port=2
  Road Gradient (rad) : Outport  Port=3
  wires:
  Road Gradient (rad)/1 -> Road Gradient (rad)/1  "Road Gradient (rad)"
  Drive Cycle Source/1 -> Velocity Profile (m/s)/1  "Velocity Profile (m/s)"
  Drive Cycle Source/2 -> Acceleration Profile (m/s^2)/1  "Acceleration Profile (m/s^2)"

== system series/Truck Force Balance/Total Mass, including Inertial Loads ==
  "Gear Ratio " : Inport
  " 1" : Gain  Gain=1/radius_wheel^2
  " 3" : Gain  Gain=momentOfInertia_engine
  Constant : Constant  Value=momentOfInertia_wheel
  Constant1 : Constant  Value=total_mass
  Square1 : Math  Operator=square  SaturateOnIntegerOverflow=on
  Sum1 : Sum  Inputs=|++
  Sum2 : Sum  Inputs=|++
  Actual Mass : Outport
  wires:
  Square1/1 -> " 3"/1
  Constant1/1 -> Sum2/2
  " 3"/1 -> Sum1/1
  Sum1/1 -> " 1"/1
  " 1"/1 -> Sum2/1
  "Gear Ratio "/1 -> Square1/1
  Constant/1 -> Sum1/2
  Sum2/1 -> Actual Mass/1

== stateflow chart series/AC induction Machine (Generator) and Controller/Engine On//Off Logic ==
  state battery [parallel]
    settings: executionOrder=2
    state discharging
    state charging
    state regenerative_braking
    (default) -> discharging
    regenerative_braking -> discharging : [regen_power == 0 || battery_SoC > 79]
    charging -> discharging : [battery_SoC > 79]
        | {engine.OFF;}
    discharging -> charging [order 2] : [battery_SoC < 25]
        | {engine.ON;}
    discharging -> regenerative_braking [order 1] : [regen_power > 0 && battery_SoC < 80]
  state engine [parallel]
    settings: executionOrder=1
    state engine_off
      entry:
      state = 0;
    state engine_on
      entry:
      state = 1;
    (default) -> engine_off
    engine_on -> engine_off : OFF
    engine_off -> engine_on : ON
  data: state output double =0; battery_SoC input double; regen_power input; engine local double
  events: ON local FUNCTION_CALL_EVENT; OFF local FUNCTION_CALL_EVENT; OFF local FUNCTION_CALL_EVENT; ON local FUNCTION_CALL_EVENT
